simulink model "LFRefMdl"  (R2020b)
settings: Solver=FixedStepDiscrete  StartTime=0.0  StopTime=inf  FixedStep=Ts  RelTol=1e-3
undefined symbols (not defined in the file): Cf, Cr, default_spacing, Iz, lag, lf, lr, m, max_ac, max_steer, min_ac, min_steer, posSelector, PredictionHorizon, tau, time_gap, Ts, v0_ego
libraries: drivinglib x2, mpclib x1
settings Model: Creator=The MathWorks, Inc.  LastModifiedBy=jferrari
settings DataIOCC: SaveOutput=off  SaveTime=off
settings OptimizationCC: DefaultParameterBehavior=Inlined  DefaultUnderspecifiedDataType=single  EnhancedBackFolding=on  PassReuseOutputArgsAs=Individual arguments  ZeroExternalMemoryAtStartup=off  ZeroInternalMemoryAtStartup=off  OptimizeBlockOrder=speed  DifferentSizesBufferReuse=on  OptimizationCustomize=off  EfficientTunableParamExpr=on
settings DebuggingCC: ParameterPrecisionLossMsg=none  ParameterTunabilityLossMsg=error  ArithmeticOperatorsInVariantConditions=warning
settings HardwareCC: ProdLongLongMode=on
settings SFSimCC: SimUseLocalCustomCode=off  MATLABDynamicMemAlloc=off  CustomCodeUndefinedFunction=UseInterfaceOnly  SimTargetLang=C++
settings RTWCC: Description=Embedded Coder  SystemTargetFile=ert.tlc  TemplateMakefile=ert_default_tmf  GenerateReport=on  RTWUseLocalCustomCode=off  BuildConfiguration=Faster Runs  IncludeHyperlinkInReport=on  LaunchReport=on  TargetLang=C++  GenerateTraceInfo=on  GenerateTraceReport=on  GenerateTraceReportSl=on  GenerateTraceReportSf=on  GenerateTraceReportEml=on  GenerateCodeMetricsReport=on
settings CodeAppCC: ForceParamTrailComments=on  IgnoreCustomStorageClasses=off  MaxIdLength=63  OperatorAnnotations=on  SimulinkDataObjDesc=on  SFDataObjDesc=on  CustomSymbolStrFcn=$N$M$F  InsertBlockDesc=on
settings ERTTargetCC: TargetLangStandard=C++03 (ISO)  GenerateSampleERTMain=on  CodeInterfacePackaging=C++ class  InlinedParameterPlacement=NonHierarchical  RootIOFormat=Structure reference  ERTCustomFileTemplate=example_file_process.tlc

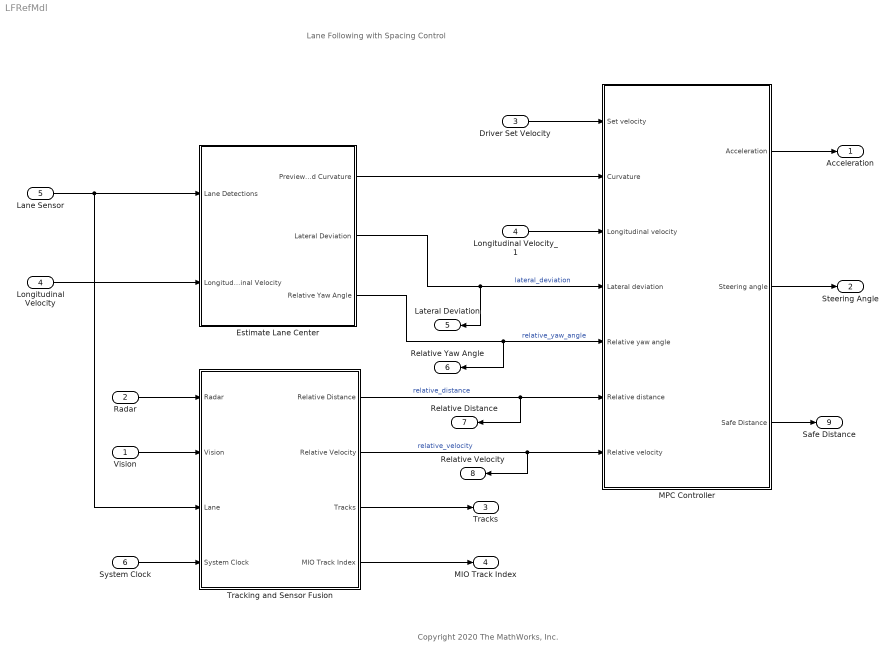
== system LFRefMdl ==
  note: Copyright 2020 The MathWorks, Inc.
  note: Lane Following with Spacing Control
  Vision : Inport  OutDataTypeStr=Bus: BusVision  PortDimensions=[1 1]  BusOutputAsStruct=on
  Radar : Inport  Port=2  OutDataTypeStr=Bus: BusRadar  PortDimensions=[1 1]  BusOutputAsStruct=on
  Driver Set Velocity : Inport  Port=3
  Longitudinal Velocity : Inport  Port=4  Unit=m/s  PortDimensions=1
  Lane Sensor : Inport  Port=5  OutDataTypeStr=Bus: LaneSensor  PortDimensions=1
  System Clock : Inport  Port=6  OutDataTypeStr=double  PortDimensions=[1 1]
  Estimate Lane Center : Subsystem  TreatAsAtomicUnit=on  VariantControl=v2
      settings: RTWFileNameOpts=Use function name
  Longitudinal Velocity_1 : InportShadow  Port=4  Unit=m/s  PortDimensions=1
  MPC Controller : Subsystem  TreatAsAtomicUnit=on  VariantControl=Variant2
      settings: RTWFileNameOpts=Use function name
  Tracking and Sensor Fusion : Subsystem  TreatAsAtomicUnit=on
      settings: RTWFileNameOpts=Use function name
  Acceleration : Outport  PortDimensions=1  VectorParamsAs1DForOutWhenUnconnected=off
  Steering Angle : Outport  Port=2  PortDimensions=1  VectorParamsAs1DForOutWhenUnconnected=off
  "Tracks " : Outport  Port=3  OutDataTypeStr=Bus:BusMultiObjectTracker1  VectorParamsAs1DForOutWhenUnconnected=off  BusOutputAsStruct=on
  MIO Track Index : Outport  Port=4  PortDimensions=1  VectorParamsAs1DForOutWhenUnconnected=off  BusOutputAsStruct=on
  Lateral Deviation : Outport  Port=5
  Relative Yaw Angle : Outport  Port=6
  Relative Distance : Outport  Port=7
  Relative Velocity : Outport  Port=8
  Safe Distance : Outport  Port=9
  wires:
  Estimate Lane Center/1(Previewed Curvature) -> MPC Controller/2(Curvature)
  Longitudinal Velocity/1 -> Estimate Lane Center/2(Longitudinal Velocity)
  Driver Set Velocity/1 -> MPC Controller/1(Set velocity)
  MPC Controller/1(Acceleration) -> Acceleration/1
  Longitudinal Velocity_1/1 -> MPC Controller/3(Longitudinal velocity)
  Estimate Lane Center/2(Lateral Deviation) -> Lateral Deviation/1, MPC Controller/4(Lateral deviation)  "lateral_deviation"
  Estimate Lane Center/3(Relative Yaw Angle) -> Relative Yaw Angle/1, MPC Controller/5(Relative yaw angle)  "relative_yaw_angle"
  Lane Sensor/1 -> Tracking and Sensor Fusion/3(Lane), Estimate Lane Center/1(Lane Detections)
  MPC Controller/2(" Steering angle") -> Steering Angle/1
  Vision/1 -> Tracking and Sensor Fusion/2(Vision)
  Radar/1 -> Tracking and Sensor Fusion/1(Radar)
  Tracking and Sensor Fusion/2(Relative Velocity) -> Relative Velocity/1, MPC Controller/7(Relative velocity)  "relative_velocity"
  Tracking and Sensor Fusion/1(Relative Distance) -> Relative Distance/1, MPC Controller/6(Relative distance)  "relative_distance"
  System Clock/1 -> Tracking and Sensor Fusion/4(System Clock)
  Tracking and Sensor Fusion/3(Tracks) -> "Tracks "/1
  Tracking and Sensor Fusion/4(MIO Track Index) -> MIO Track Index/1
  MPC Controller/3(Safe Distance) -> Safe Distance/1

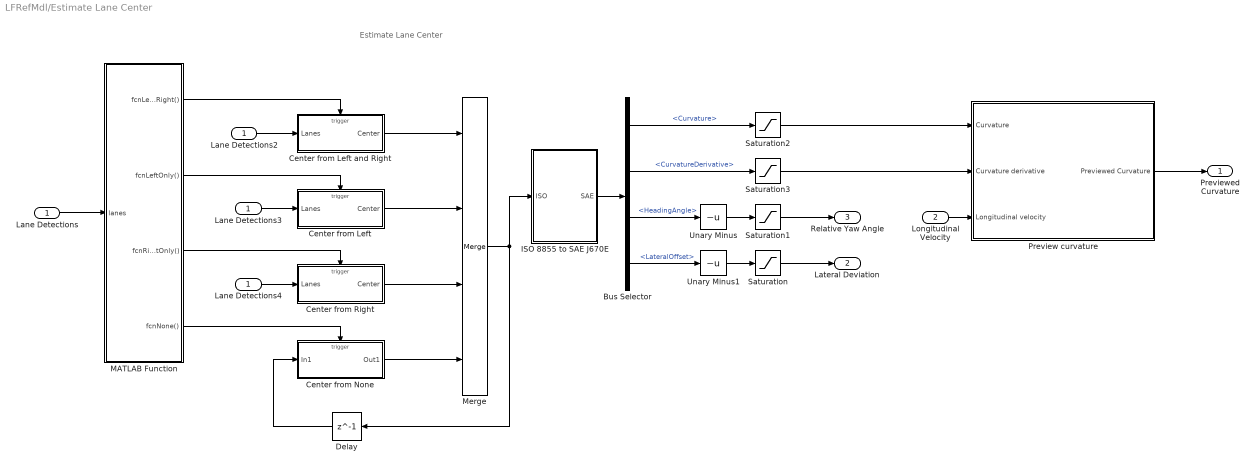
== system LFRefMdl/Estimate Lane Center ==
  note: Estimate Lane Center
  Lane Detections : Inport
  Longitudinal Velocity : Inport  Port=2
  Bus Selector : BusSelector  OutputSignals=Curvature,CurvatureDerivative,HeadingAngle,LateralOffset
  Center from Left : Subsystem  TreatAsAtomicUnit=on
  Center from Left and Right : Subsystem  TreatAsAtomicUnit=on
  Center from None : Subsystem  TreatAsAtomicUnit=on
  Center from Right : Subsystem  TreatAsAtomicUnit=on
  Delay : Delay  DelayLength=1
  ISO 8855 to SAE J670E : Subsystem
  Lane Detections2 : InportShadow
  Lane Detections3 : InportShadow
  Lane Detections4 : InportShadow
  MATLAB Function : MATLAB Function  TreatAsAtomicUnit=on
  Merge : Merge  Inputs=4
  Preview curvature : Subsystem
  Saturation : Saturate
  Saturation1 : Saturate  UpperLimit=0.6  LowerLimit=-0.6
  Saturation2 : Saturate  UpperLimit=0.15  LowerLimit=-0.15
  Saturation3 : Saturate  UpperLimit=0.06  LowerLimit=-0.06
  Unary Minus : UnaryMinus
  Unary Minus1 : UnaryMinus
  Previewed Curvature : Outport  VectorParamsAs1DForOutWhenUnconnected=off
  Lateral Deviation : Outport  Port=2  VectorParamsAs1DForOutWhenUnconnected=off
  Relative Yaw Angle : Outport  Port=3  VectorParamsAs1DForOutWhenUnconnected=off
  wires:
  Center from Right/1(Center) -> Merge/3
  Lane Detections3/1 -> Center from Left/1(Lanes)
  Lane Detections4/1 -> Center from Right/1(Lanes)
  MATLAB Function/2(fcnLeftOnly()) -> Center from Left/Trigger
  Center from None/1(Out1) -> Merge/4
  MATLAB Function/1(fcnLeftAndRight()) -> Center from Left and Right/Trigger
  Delay/1 -> Center from None/1(In1)
  Center from Left and Right/1(Center) -> Merge/1
  Lane Detections/1 -> MATLAB Function/1(lanes)
  Lane Detections2/1 -> Center from Left and Right/1(Lanes)
  MATLAB Function/3(fcnRightOnly()) -> Center from Right/Trigger
  MATLAB Function/4(fcnNone()) -> Center from None/Trigger
  Center from Left/1(Center) -> Merge/2
  Merge/1 -> ISO 8855 to SAE J670E/1(ISO), Delay/1
  Saturation3/1 -> Preview curvature/2(Curvature derivative)
  Saturation2/1 -> Preview curvature/1(Curvature)
  Saturation1/1 -> Relative Yaw Angle/1
  Saturation/1 -> Lateral Deviation/1
  Unary Minus/1 -> Saturation1/1
  Preview curvature/1(Previewed Curvature) -> Previewed Curvature/1
  Longitudinal Velocity/1 -> Preview curvature/3(Longitudinal velocity)
  Bus Selector/2 -> Saturation3/1  "<CurvatureDerivative>"
  Bus Selector/1 -> Saturation2/1  "<Curvature>"
  Unary Minus1/1 -> Saturation/1
  Bus Selector/4 -> Unary Minus1/1  "<LateralOffset>"
  Bus Selector/3 -> Unary Minus/1  "<HeadingAngle>"
  ISO 8855 to SAE J670E/1(SAE) -> Bus Selector/1

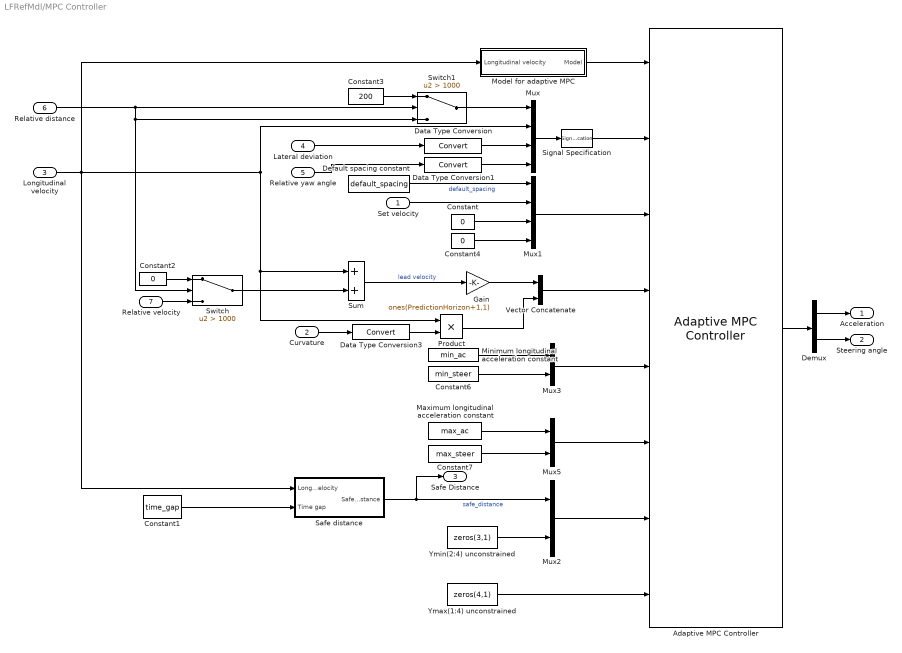
== system LFRefMdl/MPC Controller ==
  Set velocity : Inport  Unit=m/s
  Curvature : Inport  Port=2
  Longitudinal velocity : Inport  Port=3
  Lateral deviation : Inport  Port=4  Unit=m
  Relative yaw angle : Inport  Port=5  Unit=rad
  Relative distance : Inport  Port=6  Unit=m
  Relative velocity : Inport  Port=7  Unit=m/s
  Adaptive MPC Controller : mpclib/Adaptive MPC Controller  SCDEnableBlockLinearizationSpecification=on  VariantControl=Variant  mpcobj=mpc1  enable_value=0  updateMPCinCallerWorkspace=on  md_inport=on  mv_inport=off  uref_inport=off  return_cost=off  return_mvseq=off  return_qpstatus=off  return_xseq=off  return_state=off  return_ovseq=off  state_inport=off  isltv_plant=off  umin_inport=on  umax_inport=on  ymin_inport=on  ymax_inport=on  cc_inport=off  ywt_inport=off  uwt_inport=off  duwt_inport=off  rhoeps_inport=off  pm_inport=off  MaximumP=10  HorizonChoice=FixedHorizon  BlockDataType=double  SampleTimeInherited=off  switch_inport=off
  Constant : Constant  Value=0
  Constant1 : Constant  Value=time_gap  SampleTime=Ts
  Constant2 : Constant  Value=0  SampleTime=Ts
  Constant3 : Constant  Value=200  SampleTime=Ts
  Constant4 : Constant  Value=0
  Constant6 : Constant  Value=min_steer
  Constant7 : Constant  Value=max_steer
  Data Type Conversion : DataTypeConversion
  Data Type Conversion1 : DataTypeConversion
  Data Type Conversion3 : DataTypeConversion
  Default spacing constant : Constant  Value=default_spacing
  Demux : Demux  Outputs=2
  Gain : Gain  Gain=ones(PredictionHorizon+1,1)
  Maximum longitudinal acceleration constant : Constant  Value=max_ac
  Minimum longitudinal acceleration constant : Constant  Value=min_ac
  Model for adaptive MPC : Subsystem
  Mux : Mux
  Mux1 : Mux
  Mux2 : Mux  Inputs=2
  Mux3 : Mux  Inputs=2
  Mux5 : Mux  Inputs=2
  Product : Product
  Safe distance : Subsystem
  Signal Specification : SignalSpecification  Dimensions=4
  Sum : Sum
  Switch : Switch  Criteria=u2 > Threshold  Threshold=1000
  Switch1 : Switch  Criteria=u2 > Threshold  Threshold=1000
  Vector Concatenate : Concatenate  Mode=Multidimensional array  ConcatenateDimension=2
  Ymax(1:4) unconstrained : Constant  Value=zeros(4,1)  VectorParams1D=off
  Ymin(2:4) unconstrained : Constant  Value=zeros(3,1)  VectorParams1D=off
  Acceleration : Outport  Unit=m/s^2  VectorParamsAs1DForOutWhenUnconnected=off
  " Steering angle" : Outport  Port=2  Unit=rad  VectorParamsAs1DForOutWhenUnconnected=off
  Safe Distance : Outport  Port=3
  wires:
  Mux/1 -> Signal Specification/1
  Constant3/1 -> Switch1/1
  Switch1/1 -> Mux/1
  Constant2/1 -> Switch/1
  Relative velocity/1 -> Switch/3
  Switch/1 -> Sum/2
  Curvature/1 -> Data Type Conversion3/1
  Relative distance/1 -> Switch1/2, Switch/2, Switch1/3
  Set velocity/1 -> Mux1/2
  Product/1 -> Vector Concatenate/2
  Gain/1 -> Vector Concatenate/1
  Sum/1 -> Gain/1  "lead velocity"
  Relative yaw angle/1 -> Data Type Conversion1/1
  Lateral deviation/1 -> Data Type Conversion/1
  Demux/1 -> Acceleration/1
  Demux/2 -> " Steering angle"/1
  Safe distance/1(Safe distance) -> Mux2/1, Safe Distance/1  "safe_distance"
  Longitudinal velocity/1 -> Model for adaptive MPC/1(Longitudinal velocity), Safe distance/1(Longitudinal velocity), Mux/2, Sum/1, Product/1
  Constant1/1 -> Safe distance/2(Time gap)
  Default spacing constant/1 -> Mux1/1  "default_spacing"
  Minimum longitudinal acceleration constant/1 -> Mux3/1
  Constant6/1 -> Mux3/2
  Maximum longitudinal acceleration constant/1 -> Mux5/1
  Constant7/1 -> Mux5/2
  Data Type Conversion/1 -> Mux/3
  Data Type Conversion1/1 -> Mux/4
  Ymin(2:4) unconstrained/1 -> Mux2/2
  Data Type Conversion3/1 -> Product/2
  Constant/1 -> Mux1/3
  Constant4/1 -> Mux1/4
  Model for adaptive MPC/1(Model) -> Adaptive MPC Controller/1
  Signal Specification/1 -> Adaptive MPC Controller/2
  Mux1/1 -> Adaptive MPC Controller/3
  Vector Concatenate/1 -> Adaptive MPC Controller/4
  Mux3/1 -> Adaptive MPC Controller/5
  Mux5/1 -> Adaptive MPC Controller/6
  Mux2/1 -> Adaptive MPC Controller/7
  Adaptive MPC Controller/1 -> Demux/1
  Ymax(1:4) unconstrained/1 -> Adaptive MPC Controller/8

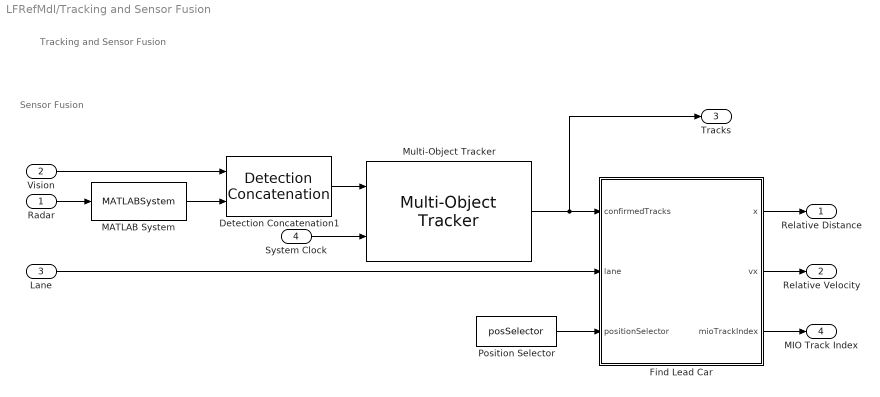
== system LFRefMdl/Tracking and Sensor Fusion ==
  note: Tracking and Sensor Fusion
  note: Sensor Fusion
  Radar : Inport  OutDataTypeStr=Bus: BusRadar  PortDimensions=[1 1]  BusOutputAsStruct=on
  Vision : Inport  Port=2  OutDataTypeStr=Bus: BusVision  PortDimensions=[1 1]  BusOutputAsStruct=on
  Lane : Inport  Port=3  OutDataTypeStr=Bus: LaneSensor  BusOutputAsStruct=on
  System Clock : Inport  Port=4  OutDataTypeStr=double  PortDimensions=[1 1]
  Detection Concatenation1 : drivinglib/Detection Concatenation  NumInputs=2  BusNameSource=Auto  BusName=BusDetectionConcatenation1  SimulateUsing=Interpreted execution
      settings: SourceProductBaseCode=DR
  Find Lead Car : MATLAB Function  TreatAsAtomicUnit=on
  MATLAB System : MATLABSystem  System=helperClusterDetections  ClusterSize=clusterSize  BusNameSource=Auto  BusName=BusClusterDetections  SimulateUsing=Interpreted execution
      mask Type: helperClusterDetections
      mask Display:
      | disp(['Detection' char(10) 'Clustering']);
      | port_label('input',1,'In');
      | port_label('output',1,'Out');
  Multi-Object Tracker : drivinglib/Multi-Object Tracker  TrackerIndex=uint32( 0 )  FilterInitializationFcn=initcvekf  AssignmentThreshold=assigThresh  ConfirmationThreshold=[ 2, 3 ]  DeletionThreshold=[ 5, 5 ]  MaxNumTracks=numTracks  MaxNumSensors=numSensors  StateParams=struct  TimeInputSource=Input port  HasCostMatrixInput=off  HasDetectableTrackIDsInput=off  BusNameSource=Property  BusName=BusMultiObjectTracker1  TentativeTracksOutputPort=off  AllTracksOutputPort=off  SimulateUsing=Interpreted execution
      settings: SourceProductBaseCode=DR
  Position Selector : Constant  Value=posSelector
  Relative Distance : Outport  VectorParamsAs1DForOutWhenUnconnected=off
  Relative Velocity : Outport  Port=2  VectorParamsAs1DForOutWhenUnconnected=off
  Tracks : Outport  Port=3  OutDataTypeStr=Bus:BusMultiObjectTracker1  PortDimensions=[1 1]  VectorParamsAs1DForOutWhenUnconnected=off  BusOutputAsStruct=on
  MIO Track Index : Outport  Port=4  VectorParamsAs1DForOutWhenUnconnected=off
  wires:
  Find Lead Car/2(vx) -> Relative Velocity/1
  Find Lead Car/3(mioTrackIndex) -> MIO Track Index/1
  Find Lead Car/1(x) -> Relative Distance/1
  Position Selector/1 -> Find Lead Car/3(positionSelector)
  Lane/1 -> Find Lead Car/2(lane)
  Detection Concatenation1/1 -> Multi-Object Tracker/1
  Multi-Object Tracker/1 -> Find Lead Car/1(confirmedTracks), Tracks/1
  Radar/1 -> MATLAB System/1
  System Clock/1 -> Multi-Object Tracker/2
  Vision/1 -> Detection Concatenation1/1
  MATLAB System/1 -> Detection Concatenation1/2

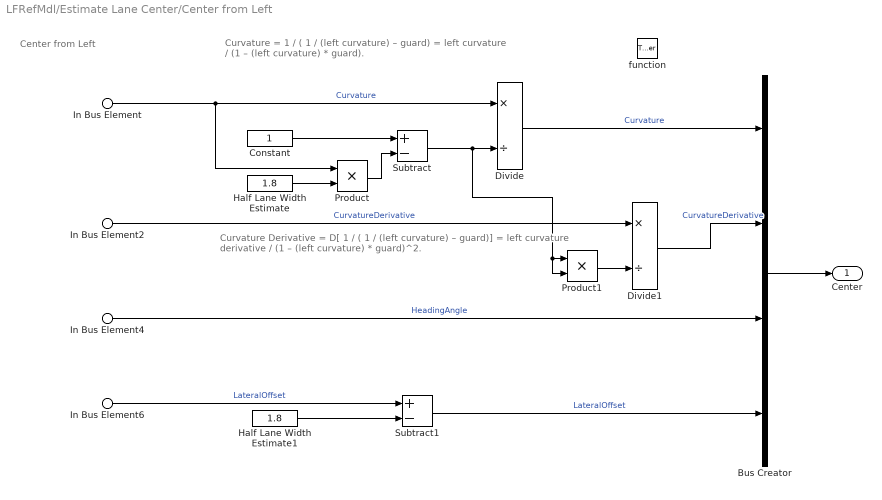
== system LFRefMdl/Estimate Lane Center/Center from Left ==
  note: Curvature Derivative
      | = D[ 1 / ( 1 / (left curvature) – guard)]
      | = left curvature derivative / (1 – (left curvature) * guard)^2.
  note: Center from Left
  note: Curvature
      | = 1 / ( 1 / (left curvature) – guard)
      | = left curvature / (1 – (left curvature) * guard).
  In Bus Element : Inport  PortName=Lanes  Element=Left.Curvature
  In Bus Element2 : Inport  PortName=Lanes  Element=Left.CurvatureDerivative
  In Bus Element4 : Inport  PortName=Lanes  Element=Left.HeadingAngle
  In Bus Element6 : Inport  PortName=Lanes  Element=Left.LateralOffset
  function : TriggerPort  TriggerType=function-call  VariantControl=Variant
  Bus Creator : BusCreator  Inputs=4
  Constant : Constant  OutDataTypeStr=Inherit: Inherit via back propagation
  Divide : Product  Inputs=*/
  Divide1 : Product  Inputs=*/
  Half Lane Width Estimate : Constant  Value=1.8  OutDataTypeStr=Inherit: Inherit via back propagation
  Half Lane Width Estimate1 : Constant  Value=1.8  OutDataTypeStr=Inherit: Inherit via back propagation
  Product : Product
  Product1 : Product
  Subtract : Sum  Inputs=+-
  Subtract1 : Sum  Inputs=+-
  Center : Outport  VectorParamsAs1DForOutWhenUnconnected=off
  wires:
  Product/1 -> Subtract/2
  Half Lane Width Estimate1/1 -> Subtract1/2
  In Bus Element6/1 -> Subtract1/1  "LateralOffset"
  Product1/1 -> Divide1/2
  In Bus Element2/1 -> Divide1/1  "CurvatureDerivative"
  Constant/1 -> Subtract/1
  Half Lane Width Estimate/1 -> Product/2
  Subtract/1 -> Divide/2, Product1/1, Product1/2
  In Bus Element/1 -> Divide/1, Product/1  "Curvature"
  Subtract1/1 -> Bus Creator/4  "LateralOffset"
  In Bus Element4/1 -> Bus Creator/3  "HeadingAngle"
  Divide/1 -> Bus Creator/1  "Curvature"
  Divide1/1 -> Bus Creator/2  "CurvatureDerivative"
  Bus Creator/1 -> Center/1

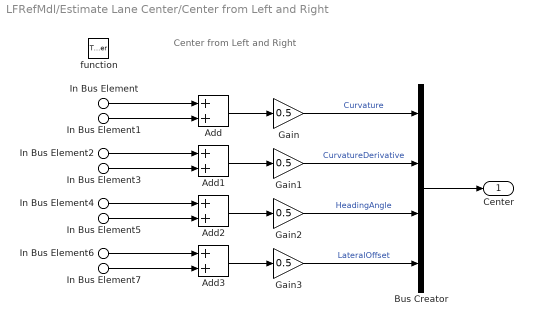
== system LFRefMdl/Estimate Lane Center/Center from Left and Right ==
  note: Center from Left and Right
  In Bus Element : Inport  PortName=Lanes  Element=Left.Curvature
  In Bus Element2 : Inport  PortName=Lanes  Element=Left.CurvatureDerivative
  In Bus Element4 : Inport  PortName=Lanes  Element=Left.HeadingAngle
  In Bus Element6 : Inport  PortName=Lanes  Element=Left.LateralOffset
  In Bus Element1 : Inport  PortName=Lanes  Element=Right.Curvature
  In Bus Element3 : Inport  PortName=Lanes  Element=Right.CurvatureDerivative
  In Bus Element5 : Inport  PortName=Lanes  Element=Right.HeadingAngle
  In Bus Element7 : Inport  PortName=Lanes  Element=Right.LateralOffset
  function : TriggerPort  TriggerType=function-call  VariantControl=Variant
  Add{,1..3} (4 alike) : Sum
  Bus Creator : BusCreator  Inputs=4
  Gain{,1..3} (4 alike) : Gain  Gain=0.5
  Center : Outport  VectorParamsAs1DForOutWhenUnconnected=off
  wires:
  In Bus Element6/1 -> Add3/1
  In Bus Element7/1 -> Add3/2
  In Bus Element5/1 -> Add2/2
  In Bus Element4/1 -> Add2/1
  In Bus Element3/1 -> Add1/2
  In Bus Element2/1 -> Add1/1
  In Bus Element1/1 -> Add/2
  In Bus Element/1 -> Add/1
  Bus Creator/1 -> Center/1
  Gain3/1 -> Bus Creator/4  "LateralOffset"
  Add3/1 -> Gain3/1
  Gain2/1 -> Bus Creator/3  "HeadingAngle"
  Add2/1 -> Gain2/1
  Gain1/1 -> Bus Creator/2  "CurvatureDerivative"
  Add1/1 -> Gain1/1
  Gain/1 -> Bus Creator/1  "Curvature"
  Add/1 -> Gain/1

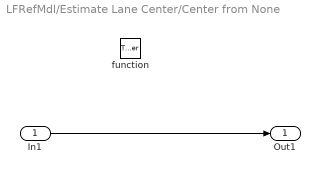
== system LFRefMdl/Estimate Lane Center/Center from None ==
  In1 : Inport
  function : TriggerPort  TriggerType=function-call  VariantControl=Variant
  Out1 : Outport  VectorParamsAs1DForOutWhenUnconnected=off
  wires:
  In1/1 -> Out1/1

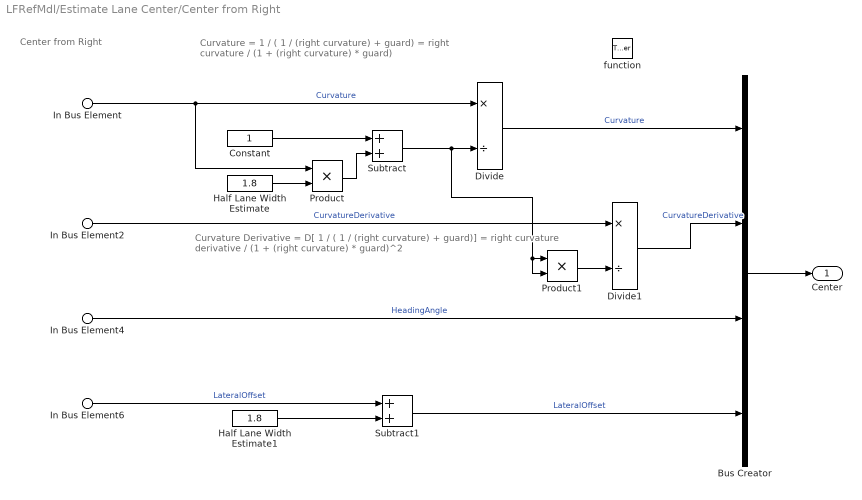
== system LFRefMdl/Estimate Lane Center/Center from Right ==
  note: Curvature Derivative
      | = D[ 1 / ( 1 / (right curvature) + guard)]
      | = right curvature derivative / (1 + (right curvature) * guard)^2
  note: Curvature
      | = 1 / ( 1 / (right curvature) + guard)
      | = right curvature / (1 + (right curvature) * guard)
  note: Center from Right
  In Bus Element : Inport  PortName=Lanes  Element=Right.Curvature
  In Bus Element2 : Inport  PortName=Lanes  Element=Right.CurvatureDerivative
  In Bus Element4 : Inport  PortName=Lanes  Element=Right.HeadingAngle
  In Bus Element6 : Inport  PortName=Lanes  Element=Right.LateralOffset
  function : TriggerPort  TriggerType=function-call  VariantControl=Variant
  Bus Creator : BusCreator  Inputs=4
  Constant : Constant  OutDataTypeStr=Inherit: Inherit via back propagation
  Divide : Product  Inputs=*/
  Divide1 : Product  Inputs=*/
  Half Lane Width Estimate : Constant  Value=1.8  OutDataTypeStr=Inherit: Inherit via back propagation
  Half Lane Width Estimate1 : Constant  Value=1.8  OutDataTypeStr=Inherit: Inherit via back propagation
  Product : Product
  Product1 : Product
  Subtract : Sum
  Subtract1 : Sum
  Center : Outport  VectorParamsAs1DForOutWhenUnconnected=off
  wires:
  Half Lane Width Estimate/1 -> Product/2
  Product/1 -> Subtract/2
  Constant/1 -> Subtract/1
  Subtract/1 -> Divide/2, Product1/1, Product1/2
  In Bus Element/1 -> Divide/1, Product/1  "Curvature"
  Bus Creator/1 -> Center/1
  Subtract1/1 -> Bus Creator/4  "LateralOffset"
  Divide/1 -> Bus Creator/1  "Curvature"
  In Bus Element6/1 -> Subtract1/1  "LateralOffset"
  Half Lane Width Estimate1/1 -> Subtract1/2
  In Bus Element4/1 -> Bus Creator/3  "HeadingAngle"
  Product1/1 -> Divide1/2
  Divide1/1 -> Bus Creator/2  "CurvatureDerivative"
  In Bus Element2/1 -> Divide1/1  "CurvatureDerivative"

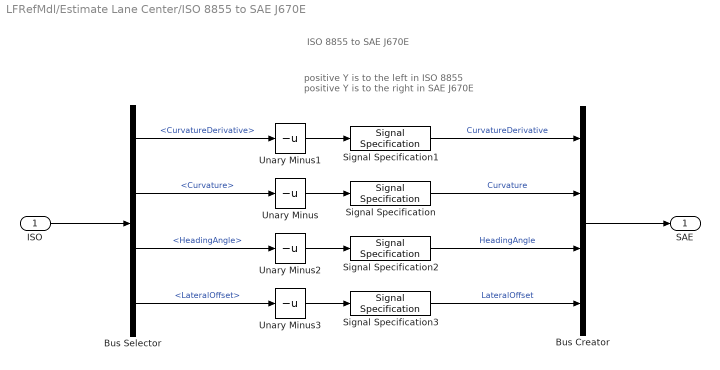
== system LFRefMdl/Estimate Lane Center/ISO 8855 to SAE J670E ==
  note: positive Y is to the left in ISO 8855
      | positive Y is to the right in SAE J670E
  note: ISO 8855 to SAE J670E
  ISO : Inport
  Bus Creator : BusCreator  Inputs=4
  Bus Selector : BusSelector  OutputSignals=CurvatureDerivative,Curvature,HeadingAngle,LateralOffset
  Signal Specification : SignalSpecification  Unit=1/m^2
  Signal Specification1 : SignalSpecification  Unit=1/m
  Signal Specification2 : SignalSpecification  Unit=rad
  Signal Specification3 : SignalSpecification  Unit=m
  Unary Minus{,1..3} (4 alike) : UnaryMinus
  SAE : Outport  VectorParamsAs1DForOutWhenUnconnected=off
  wires:
  ISO/1 -> Bus Selector/1
  Bus Selector/2 -> Unary Minus/1  "<Curvature>"
  Bus Selector/1 -> Unary Minus1/1  "<CurvatureDerivative>"
  Bus Selector/3 -> Unary Minus2/1  "<HeadingAngle>"
  Bus Selector/4 -> Unary Minus3/1  "<LateralOffset>"
  Bus Creator/1 -> SAE/1
  Signal Specification/1 -> Bus Creator/2  "Curvature"
  Unary Minus1/1 -> Signal Specification1/1
  Unary Minus2/1 -> Signal Specification2/1
  Unary Minus3/1 -> Signal Specification3/1
  Unary Minus/1 -> Signal Specification/1
  Signal Specification1/1 -> Bus Creator/1  "CurvatureDerivative"
  Signal Specification2/1 -> Bus Creator/3  "HeadingAngle"
  Signal Specification3/1 -> Bus Creator/4  "LateralOffset"

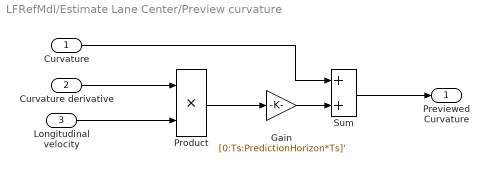
== system LFRefMdl/Estimate Lane Center/Preview curvature ==
  Curvature : Inport
  Curvature derivative : Inport  Port=2
  Longitudinal velocity : Inport  Port=3
  Gain : Gain  Gain=[0:Ts:PredictionHorizon*Ts]'
  Product : Product
  Sum : Sum
  Previewed Curvature : Outport  VectorParamsAs1DForOutWhenUnconnected=off
  wires:
  Sum/1 -> Previewed Curvature/1
  Curvature/1 -> Sum/1
  Gain/1 -> Sum/2
  Product/1 -> Gain/1
  Longitudinal velocity/1 -> Product/2
  Curvature derivative/1 -> Product/1

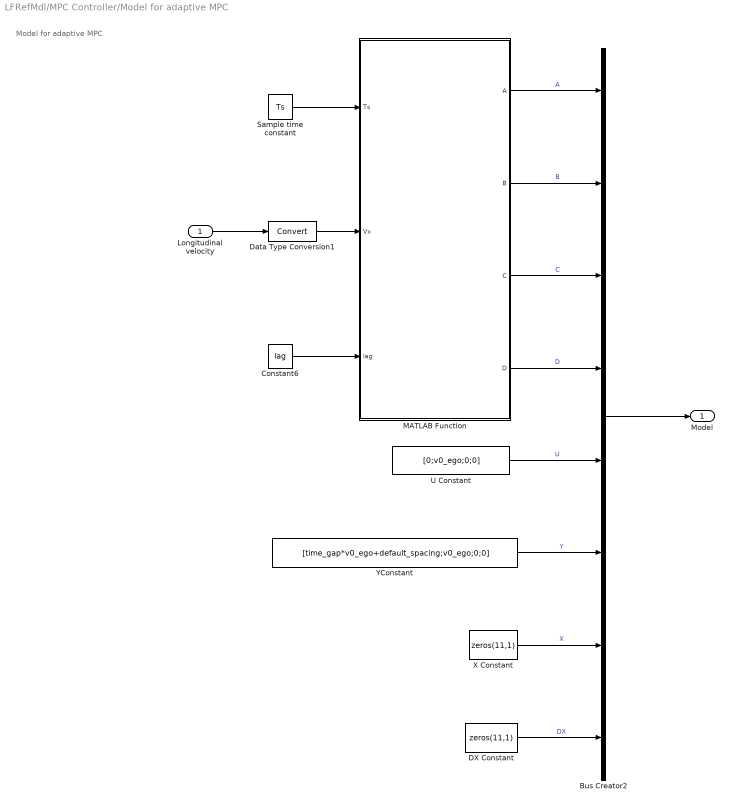
== system LFRefMdl/MPC Controller/Model for adaptive MPC ==
  note: Model for adaptive MPC
  Longitudinal velocity : Inport
  Bus Creator2 : BusCreator  Inputs=8
  Constant6 : Constant  Value=lag
  DX Constant : Constant  Value=zeros(11,1)  VectorParams1D=off
  Data Type Conversion1 : DataTypeConversion
  MATLAB Function : MATLAB Function  TreatAsAtomicUnit=on
  Sample time constant : Constant  Value=Ts
  U Constant : Constant  Value=[0;v0_ego;0;0]  VectorParams1D=off
  X Constant : Constant  Value=zeros(11,1)  VectorParams1D=off
  YConstant : Constant  Value=[time_gap*v0_ego+default_spacing;v0_ego;0;0]  VectorParams1D=off
  Model : Outport  VectorParamsAs1DForOutWhenUnconnected=off
  wires:
  MATLAB Function/4(D) -> Bus Creator2/4  "D"
  X Constant/1 -> Bus Creator2/7  "X"
  Bus Creator2/1 -> Model/1
  Longitudinal velocity/1 -> Data Type Conversion1/1
  Sample time constant/1 -> MATLAB Function/1(Ts)
  MATLAB Function/1(A) -> Bus Creator2/1  "A"
  DX Constant/1 -> Bus Creator2/8  "DX"
  MATLAB Function/2(B) -> Bus Creator2/2  "B"
  MATLAB Function/3(C) -> Bus Creator2/3  "C"
  Data Type Conversion1/1 -> MATLAB Function/2(Vx)
  Constant6/1 -> MATLAB Function/3(lag)
  YConstant/1 -> Bus Creator2/6  "Y"
  U Constant/1 -> Bus Creator2/5  "U"

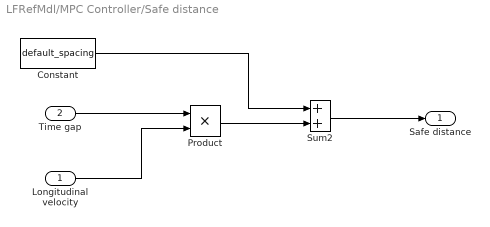
== system LFRefMdl/MPC Controller/Safe distance ==
  Longitudinal velocity : Inport
  Time gap : Inport  Port=2
  Constant : Constant  Value=default_spacing  SampleTime=Ts
  Product : Product
  Sum2 : Sum
  Safe distance : Outport  VectorParamsAs1DForOutWhenUnconnected=off
  wires:
  Sum2/1 -> Safe distance/1
  Constant/1 -> Sum2/1
  Time gap/1 -> Product/1
  Longitudinal velocity/1 -> Product/2
  Product/1 -> Sum2/2

== matlab function LFRefMdl/MPC Controller/Model for adaptive MPC/MATLAB Function ==
  data: Ts input; A output; Vx input; B output; C output; D output; lag input; tau parameter; m parameter; Cr parameter; Cf parameter; lr parameter; lf parameter; Iz parameter
function [A,B,C,D] = getAdaptiveMPCModel(Ts,Vx,lag,tau,m, Cr, Cf, lr, lf, Iz)
% Get discrete state-space model for Adaptive MPC with sample time Ts.

% Inputs:
%   Ts:               sample time
%   Vx:               longitudinal velocity
%   Ag,Bg,Cg:         continuous vehicle lateral model  
%   lag:              lumped lag caused by actuator, sensor, communication delays
% Outputs:
%   A,B,C,D:          discrete time model for adaptive MPC

%   Author: Meng Xia, Rong Chen
%   Copyright 2017-2018 The MathWorks, Inc.

% Discrete MPC model
[A,B,C,D] = getDiscreteModelForAdaptiveMPC(Ts,Vx,lag,tau,m, Cr, Cf, lr, lf, Iz);

== matlab function LFRefMdl/Tracking and Sensor Fusion/Find Lead Car ==
  data: confirmedTracks input; x output size=[1 1]; vx output size=[1 1]; lane input; mioTrackIndex output; positionSelector input
function [x,vx,mioTrackIndex] = findLeadCar(confirmedTracks, lane, positionSelector)
% This function finds the lead car: a car in front of the ego car that
% satisfies all the criteria below:
% * Within the ego car's lane.
% * In front of the ego car.
% * Closest to the ego car.

% Note: If you change state definition, change the following:
%       State = [x;vx;y;vy;z;vz] (3D constant velocity)
numStates = 6;

% Initialize outputs and parameters
maxX = cast(1000, 'like', confirmedTracks.Tracks(1).State);  % Far enough forward so that no track is expected to exceed this distance
mioTrackIndex = 0;

% If lane detection is not available, the ego car is assumed to be located
% in the middle of its lane. The lane width is assumed to be 3.6m, typical
% highway lane width.
laneWidth = 3.6;
halfLaneWidth = laneWidth/2;

if lane.Left.Strength > 0.01
    lb = [lane.Left.CurvatureDerivative/6,...
        lane.Left.Curvature/2,...
        lane.Left.HeadingAngle,...
        lane.Left.LateralOffset];
else
    lb = single([0,0,0,halfLaneWidth]);
end

if lane.Right.Strength > 0.01
    rb = [lane.Right.CurvatureDerivative/6,...
        lane.Right.Curvature/2,...
        lane.Right.HeadingAngle,...
        lane.Right.LateralOffset];
else
    rb = single([0,0,0,-halfLaneWidth]);    
end

for i = 1:confirmedTracks.NumTracks
    position = positionSelector * confirmedTracks.Tracks(i).State;
    x = position(1); % Longitudinal position of the track relative to ego
    y = position(2); % Lateral position of the track relative to ego
    
    if x < maxX && x > 0 % No point checking otherwise

        yleftLane  = polyval(lb,x); % lateral position of left lane
        yrightLane = polyval(rb,x); % lateral position of right lane
        
        % Find a new lead car
        if (yrightLane <= y) && (y <= yleftLane)
            maxX = x;
            mioTrackIndex(:) = i;
        end
    end
end

if mioTrackIndex>0
    mioState = confirmedTracks.Tracks(mioTrackIndex).State;
else
    mioState = inf(numStates,1,'like',confirmedTracks.Tracks(1).State);
end

% Output:
x = mioState(1);    % Longitudinal position of the lead car
vx = mioState(2);   % Longitudinal velocity of the lead car

== matlab function LFRefMdl/Estimate Lane Center/MATLAB Function ==
  data: lanes input
  events: fcnLeftAndRight output FUNCTION_CALL_EVENT; fcnLeftOnly output FUNCTION_CALL_EVENT; fcnRightOnly output FUNCTION_CALL_EVENT; fcnNone output FUNCTION_CALL_EVENT
function fcn(lanes)

leftStrength  = lanes.Left.Strength;
rightStrength = lanes.Right.Strength;

if (leftStrength > 0) && (rightStrength > 0)
   fcnLeftAndRight();
   
elseif leftStrength > 0
    fcnLeftOnly();
    
elseif rightStrength > 0
    fcnRightOnly();
    
else
    fcnNone();
end
